simulink model "Q4_load_added_truck"  (R2024b)
settings: Solver=VariableStepAuto  StartTime=0.0  StopTime=100  RelTol=1e-3
model workspace (MAT data in the model file):
  F = 20
  K1 = 80
  K2 = 500
  Mt = 200
  Mv = 2500
  b1 = 350
  b2 = 15020
settings Model: Creator=chall  LastModifiedBy=chall

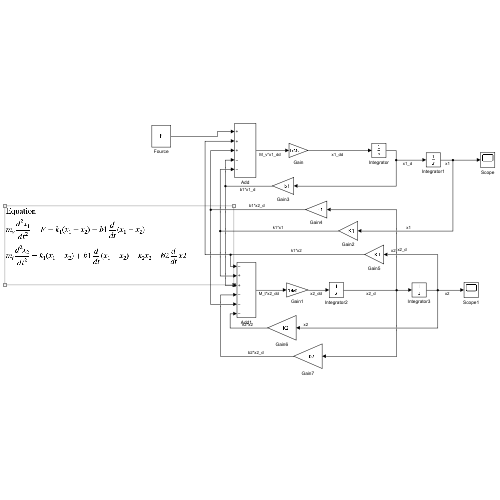
[thumbnail: Simulink's stored preview of the top-level diagram]
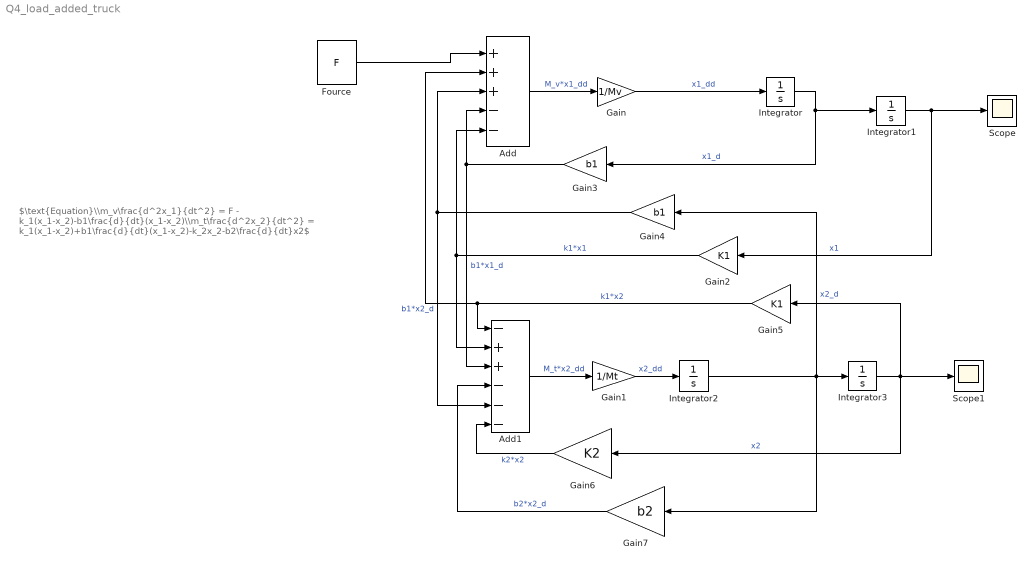
== system Q4_load_added_truck ==
  note: $\text{Equation}\\m_v\frac{d^2x_1}{dt^2} = F - k_1(x_1-x_2)-b1\frac{d}{dt}(x_1-x_2)\\m_t\frac{d^2x_2}{dt^2} = k_1(x_1-x_2)+b1\frac{d}{dt}(x_1-x_2)-k_2x_2-b2\frac{d}{dt}x2$
  Add : Sum  Inputs=+++--
  Add1 : Sum  Inputs=-++---
  Fource : Constant  Value=F
  Gain : Gain  Gain=1/Mv
  Gain1 : Gain  Gain=1/Mt
  Gain2 : Gain  Gain=K1
  Gain3 : Gain  Gain=b1
  Gain4 : Gain  Gain=b1
  Gain5 : Gain  Gain=K1
  Gain6 : Gain  Gain=K2
  Gain7 : Gain  Gain=b2
  Integrator{,1..3} (4 alike) : Integrator
  Scope : Scope
  Scope1 : Scope
  wires:
  Add/1 -> Gain/1  "M_v*x1_dd"
  Gain/1 -> Integrator/1  "x1_dd"
  Integrator/1 -> Gain3/1, Integrator1/1  "x1_d"
  Integrator1/1 -> Scope/1, Gain2/1  "x1"
  Add1/1 -> Gain1/1  "M_t*x2_dd"
  Gain1/1 -> Integrator2/1  "x2_dd"
  Integrator2/1 -> Gain4/1, Integrator3/1, Gain7/1  "x2_d"
  Integrator3/1 -> Gain5/1, Scope1/1, Gain6/1  "x2"
  Gain2/1 -> Add1/2, Add/5  "k1*x1"
  Fource/1 -> Add/1
  Gain3/1 -> Add1/3, Add/4  "b1*x1_d"
  Gain4/1 -> Add1/5, Add/3  "b1*x2_d"
  Gain5/1 -> Add1/1, Add/2  "k1*x2"
  Gain6/1 -> Add1/6  "k2*x2"
  Gain7/1 -> Add1/4  "b2*x2_d"
